simulink model "model01"  (R2021a)
settings: Solver=VariableStepAuto  StartTime=0  StopTime=tf  RelTol=1e-3
model workspace (MAT data in the model file):
  G0 = [0.005; 0.00070738]
  QSOFC = 1
  T0 = [287.15; 287.15; 287.15; 287.15]
  Tw = 10
  Tw_SOFC = 283.15
  flow_Q = 0
  hour0 = 1
values from neighbouring files (symbols this model uses):
  area = 0.01    [create_p.mat]    (also in create_params.m; model01_simulation_loop.m = 150)
  clima = clima_fcn(posixtime(dat_time))    [model01_simulation_loop.m]    (also in model_compile.m = [273.15+10 400 50 0.1])
  cp_H2O = 4182    [create_p.mat]    (also in create_params.m; model01_simulation_loop.m)
  l_w = 0.01    [create_p.mat]    (also in create_params.m; model01_simulation_loop.m)
  lamb_s = 2    [create_p.mat]    (also in create_params.m; model01_simulation_loop.m)
  mtotal = 10    [create_p.mat]    (also in create_params.m; model01_simulation_loop.m = 100)
libraries: HORTISIM x6
settings Model: SimulationMode=accelerator  ParameterArgumentNames=Tw  OrderedModelArguments=off  Creator=djoroya  LastModifiedBy=djoroya
settings DataIOCC: SaveFormat=StructureWithTime
settings OptimizationCC: EfficientMapNaN2IntZero=off
settings DebuggingCC: UnconnectedInputMsg=none  UnconnectedOutputMsg=none  UnconnectedLineMsg=none
settings HardwareCC: TargetBitPerLong=64  TargetBitPerPointer=64  TargetBitPerSizeT=64  TargetBitPerPtrDiffT=64  TargetLongLongMode=on  TargetIntDivRoundTo=Zero  TargetEndianess=LittleEndian  TargetWordSize=64  TargetHWDeviceType=MATLAB Host  ProdEqTarget=off
settings CodeAppCC: MaxIdLength=128
settings GRTTargetCC: GRTInterface=on

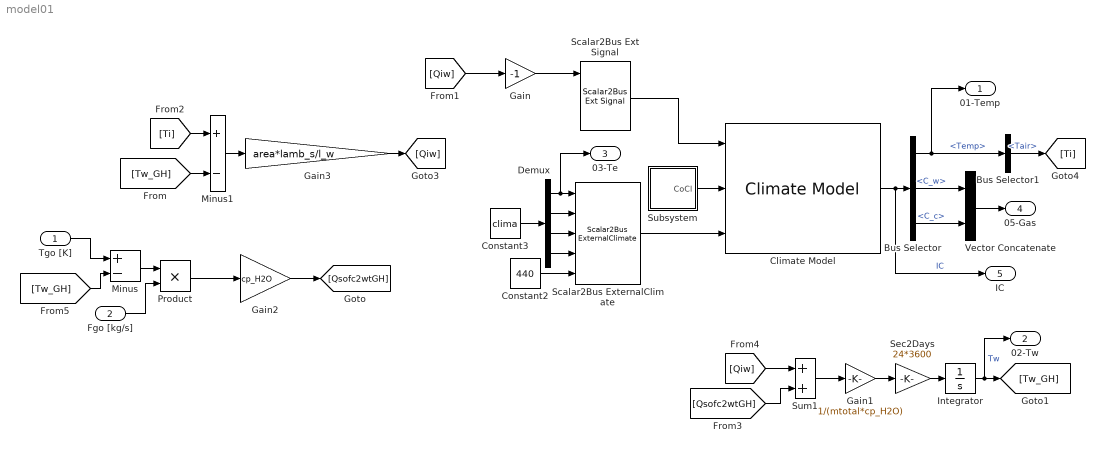
== system model01 ==
  Tgo [K] : Inport
  Fgo [kg/s] : Inport  Port=2
  Bus Selector : BusSelector  OutputSignals=Temp,Gas.C_w,Gas.C_c
  Bus Selector1 : BusSelector  OutputSignals=Tair
  Climate Model : HORTISIM/Climate/Models/Climate Model  hour0=hour0  G0=G0  T0=T0  H=climate_GH3.H  A_f=climate_GH3.A_f  A_c=climate_GH3.A_c  minWindows=climate_GH3.minWindows  lam_s=climate_GH3.lam_s  c_s=climate_GH3.c_s  l_s=climate_GH3.l_s  rhod_s=climate_GH3.rhod_s  int_air_speed=climate_GH3.int_air_speed  alpha_i=climate_GH3.alpha_i  alpha_c=climate_GH3.alpha_c  tau_c=climate_GH3.tau_c  alpha_f=climate_GH3.alpha_f  d_c=climate_GH3.d_c  cd_c=climate_GH3.cd_c  T_ss=climate_GH3.T_ss
      settings: SourceProductName=Horti Simulator
  Constant2 : Constant  Value=440
  Constant3 : Constant  Value=clima
  Demux : Demux
  Gain : Gain  Gain=-1
  Gain1 : Gain  Gain=1/(mtotal*cp_H2O)
  Gain2 : Gain  Gain=cp_H2O
  Gain3 : Gain  Gain=area*lamb_s/l_w
  Integrator : Integrator  InitialCondition=Tw
  Minus : Sum  Inputs=+-
  Minus1 : Sum  Inputs=+-
  Product : Product
  "Scalar2Bus Ext Signal " : HORTISIM/Other  Functions/Scalar2Bus Ext Signal    SystemSampleTime=-1  VariantActivationTime=update diagram  Latency=0  AutoFrameSizeCalculation=off
      settings: SourceProductName=Horti Simulator
  Scalar2Bus ExternalClimate : HORTISIM/Other  Functions/Scalar2Bus ExternalClimate  SystemSampleTime=-1  VariantActivationTime=update diagram  Latency=0  AutoFrameSizeCalculation=off
      settings: SourceProductName=Horti Simulator
  Sec2Days : Gain  Gain=24*3600
  Subsystem : Subsystem
  Sum1 : Sum
  Vector Concatenate : Concatenate
  01-Temp : Outport
  02-Tw : Outport  Port=2
  03-Te : Outport  Port=3
  05-Gas : Outport  Port=4
  IC : Outport  Port=5
  wires:
  Integrator/1 -> 02-Tw/1, [Tw_GH]  "Tw"
  Sum1/1 -> Gain1/1
  [Ti] -> Minus1/1
  [Tw_GH] -> Minus1/2
  [Qiw] -> Sum1/1
  Subsystem/1(CoCl) -> Climate Model/2
  Climate Model/1 -> IC/1, Bus Selector/1  "IC"
  Scalar2Bus ExternalClimate/1 -> Climate Model/3
  Constant2/1 -> Scalar2Bus ExternalClimate/5
  Bus Selector/1 -> Bus Selector1/1, 01-Temp/1  "<Temp>"
  Constant3/1 -> Demux/1
  Demux/3 -> Scalar2Bus ExternalClimate/3
  Demux/2 -> Scalar2Bus ExternalClimate/2
  Demux/1 -> 03-Te/1, Scalar2Bus ExternalClimate/1
  Demux/4 -> Scalar2Bus ExternalClimate/4
  Gain/1 -> "Scalar2Bus Ext Signal "/1
  "Scalar2Bus Ext Signal "/1 -> Climate Model/1
  [Qiw] -> Gain/1
  Gain1/1 -> Sec2Days/1
  Sec2Days/1 -> Integrator/1
  Bus Selector1/1 -> [Ti]  "<Tair>"
  Bus Selector/2 -> Vector Concatenate/1  "<C_w>"
  Bus Selector/3 -> Vector Concatenate/2  "<C_c>"
  Vector Concatenate/1 -> 05-Gas/1
  Minus1/1 -> Gain3/1
  Gain3/1 -> [Qiw]
  [Qsofc2wtGH] -> Sum1/2
  Tgo [K]/1 -> Minus/1
  [Tw_GH] -> Minus/2
  Minus/1 -> Product/1
  Fgo [kg/s]/1 -> Product/2
  Gain2/1 -> [Qsofc2wtGH]
  Product/1 -> Gain2/1

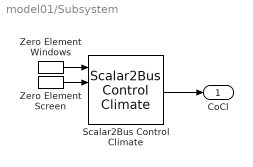
== system model01/Subsystem ==
  Scalar2Bus Control Climate : HORTISIM/Other  Functions/Scalar2Bus  Control Climate  SystemSampleTime=-1  VariantActivationTime=update diagram  Latency=0  AutoFrameSizeCalculation=off
      settings: SourceProductName=Horti Simulator
  Zero Element Screen : HORTISIM/Other  Functions/Zero Element Screen  SystemSampleTime=-1  VariantActivationTime=update diagram  Latency=0  AutoFrameSizeCalculation=off
      settings: SourceProductName=Horti Simulator
  Zero Element Windows : HORTISIM/Other  Functions/Zero Element Windows  SystemSampleTime=-1  VariantActivationTime=update diagram  Latency=0  AutoFrameSizeCalculation=off
      settings: SourceProductName=Horti Simulator
  CoCl : Outport
  wires:
  Scalar2Bus Control Climate/1 -> CoCl/1
  Zero Element Windows/1 -> Scalar2Bus Control Climate/1
  Zero Element Screen/1 -> Scalar2Bus Control Climate/2
